simulink model "nid_cvst_corner_detection"  (Simulink 7.8)
settings: Solver=FixedStepDiscrete  StartTime=0.0  StopTime=inf  RelTol=1e-3
undefined symbols (not defined in the file or in its folder): fspecial, Rec, SDTV
libraries: nid_lib x3, visionconversions x2, visionsinks x2, visionanalysis x1, visiontextngfix x1
settings Model: Creator=nmaeda  LastModifiedBy=tchikama
settings OptimizationCC: SimCompilerOptimization=On
settings DebuggingCC: InheritedTsInSrcMsg=none  ParameterPrecisionLossMsg=none
settings RTWCC: RTWCompilerOptimization=On

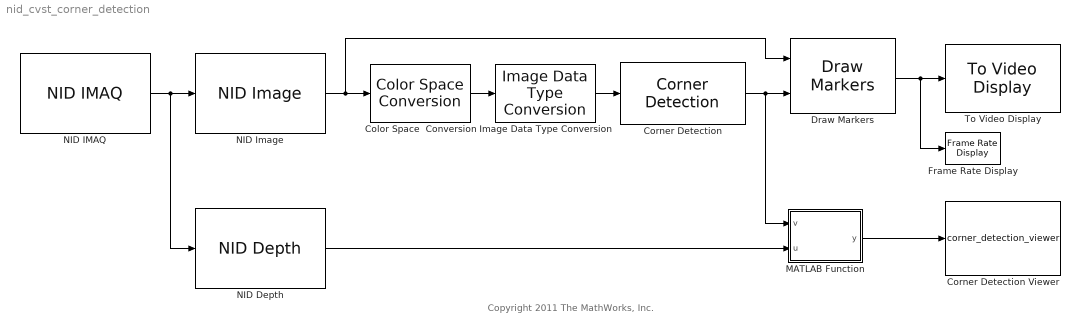
== system nid_cvst_corner_detection ==
  note: Copyright 2011 The MathWorks, Inc.
  Color Space  Conversion : visionconversions/Color Space  Conversion  conversion=Obsolete  conversionActive=R'G'B' to intensity  wp_str=D65  rec=Rec. 601 (SDTV)  sys=1125/60/2:1  imagePorts=One multidimensional signal
  Corner Detection : visionanalysis/Corner Detection  method=Local intensity comparison (Rosen & Drummond)  factor=0.1  filter=fspecial('gaussian', [1 5], 1.5)  thrInten=0.25  thrAngle=112.5  output=Obsolete9b  outputInUse=Corner location  maxNum=32  thrMetric=0.001  neighborSize=[21 21]  isOutVarDim=on  accumMode=Binary point scaling  accumWordLength=32  accumFracLength=0  prodOutputMode=Binary point scaling  prodOutputWordLength=32  prodOutputFracLength=0  memoryMode=Binary point scaling  memoryWordLength=32  memoryFracLength=0  firstCoeffMode=Specify word length  firstCoeffWordLength=16  firstCoeffFracLength=16  roundingMode=Floor  overflowMode=off
  Corner Detection Viewer : M-S-Function  FunctionName=corner_detection_viewer
      mask Display:
      | disp('Corner\nDetection\nViewer')
      | 
      | port_label('input', 1, 'XYZ')
  Draw Markers : visiontextngfix/Draw Markers  shape=Circle  size=3  fill=on  fillClrSource=Specify via dialog  display=User-specified value  intensity=200  color=[200 255 100]  opacity=0.6  viewport=Entire image  antialiasing=off  inType=Obsolete  imagePorts=One multidimensional signal  prodOutputMode=Binary point scaling  prodOutputWordLength=32  prodOutputFracLength=14  memoryMode=Specify word length  memoryWordLength=16  memoryFracLength=14  roundingMode=Floor  overflowMode=off
  Frame Rate Display : visionsinks/Frame Rate Display  UpdateRate=10
  Image Data Type Conversion : visionconversions/Image Data Type Conversion  outDT=single  isSigned=on  wordLen=16  numFracBits=0
  MATLAB Function : MATLAB Function  TreatAsAtomicUnit=on
  NID Depth : nid_lib/NID Depth  depthOutput=XYZ  conv_XYZ_RW=on  viewer=off
  NID IMAQ : nid_lib/NID IMAQ  imaq_depth=on  imaq_motion=off  imaq_image=on  view_point=on  imaq_skeleton=off  imaq_ir=off  mirror_image=off  res_fps=VGA (640x480): 30 FPS  imaq_sample_time=1/30
  NID Image : nid_lib/NID Image  imageOutput=RGB
  To Video Display : visionsinks/To Video Display  inputType=Obsolete  imagePorts=One multidimensional signal  OutputDevice=On-screen video monitor  fullScreen=off  videoWindowX=55  videoWindowY=16  saveWindowSize=off  videoWindowWidth=320  videoWindowHeight=240  dataOrg=Column-major  openAtMdlStart=on  isWindowOpen=off  inputColorFormat=RGB
  wires:
  NID IMAQ/1 -> NID Image/1, NID Depth/1
  Draw Markers/1 -> To Video Display/1, Frame Rate Display/1
  NID Image/1 -> Color Space  Conversion/1, Draw Markers/1
  Color Space  Conversion/1 -> Image Data Type Conversion/1
  Image Data Type Conversion/1 -> Corner Detection/1
  Corner Detection/1 -> Draw Markers/2, MATLAB Function/1(v)
  NID Depth/1 -> MATLAB Function/2(u)
  MATLAB Function/1(y) -> Corner Detection Viewer/1

== matlab function MATLAB Function ==
  data: v input double size=[32 2]; u input double; y output double size=[32 3]
function y = fcn(v,u)
%#codegen

n = size(v,1);
coder.varsize('tmp',[32,3]);

tmp = zeros(32,3,'double');

for i = 1:n
    tmp(i,1) = double(u(v(i,2), v(i,1), 1));
    tmp(i,2) = double(u(v(i,2), v(i,1), 2));
    tmp(i,3) = double(u(v(i,2), v(i,1), 3));
end

y = tmp;
